simulink model "transystem2_testcase_5"  (R2019b)
settings: Solver=ode15s  StartTime=0.0  StopTime=1  RelTol=1e-3  AbsTol=1e-6
libraries: powerlib x48
settings Model: ExtModeTrigMode=oneshot  ExtModeArmWhenConnect=off  Creator=Dr. Lotfifard  LastModifiedBy=RAMYA
settings SolverCC: AutoScaleAbsTol=off
settings DataIOCC: SaveFormat=Array  SignalLoggingSaveFormat=ModelDataLogs  ReturnWorkspaceOutputs=off
settings OptimizationCC: BlockReduction=off  BooleanDataType=off  ExpressionDepthLimit=2147483647  LifeSpan=inf
settings DebuggingCC: SaveWithParameterizedLinksMsg=none  UnderspecifiedInitializationDetection=Classic  MergeDetectMultiDrivingBlocksExec=none  SignalResolutionControl=TryResolveAllWithWarning  MultiTaskDSMMsg=warning  MultiTaskCondExecSysMsg=none  FcnCallInpInsideContextMsg=warning  StateNameClashWarn=warning  SFUnexpectedBacktrackingDiag=warning  SFNoUnconditionalDefaultTransitionDiag=warning  SFExecutionAtInitializationDiag=none  ArithmeticOperatorsInVariantConditions=warning
settings HardwareCC: ProdBitPerPointer=32  ProdBitPerSizeT=32  ProdBitPerPtrDiffT=32  ProdLargestAtomicFloat=None  ProdIntDivRoundTo=Undefined  ProdEndianess=Unspecified  ProdWordSize=32  ProdHWDeviceType=32-bit Generic  TargetUnknown=on
settings ModelReferenceCC: PropagateSignalLabelsOutOfModel=off
settings SFSimCC: SimUseLocalCustomCode=off  CustomCodeUndefinedFunction=UseInterfaceOnly
settings RTWCC: RTWUseLocalCustomCode=off
settings CodeAppCC: StateflowObjectComments=on
settings GRTTargetCC: TargetLangStandard=C89/C90 (ANSI)  GeneratePreprocessorConditionals=Disable all  CombineOutputUpdateFcns=off  GRTInterface=on
settings ConfigComp: CovMetricSettings=dw  CovHtmlReporting=on  CovSaveCumulativeToWorkspaceVar=on  CovSaveSingleToWorkspaceVar=on  CovExternalEMLEnable=off
settings SimscapeCC: SimscapeNormalizeSystem=off

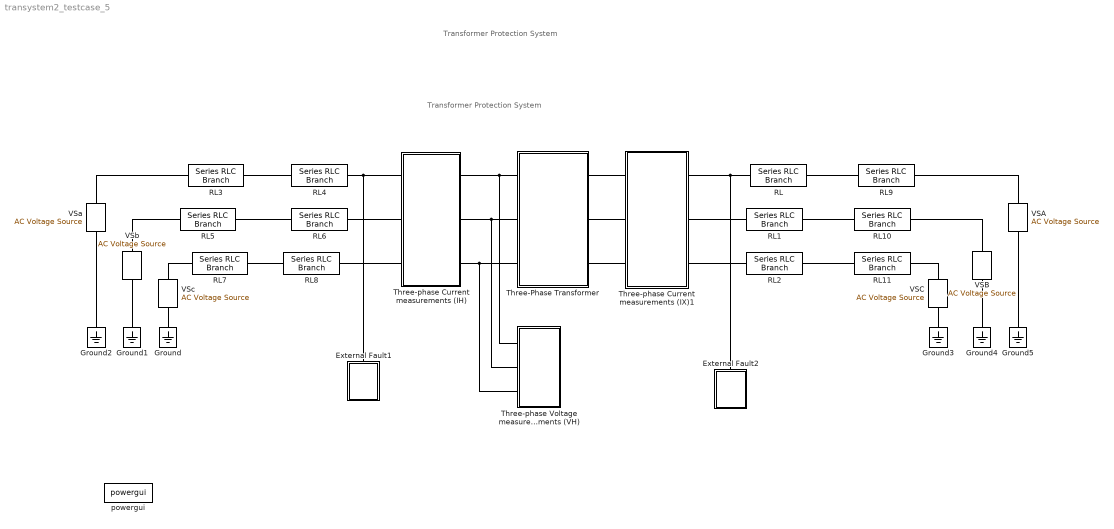
== system transystem2_testcase_5 ==
  note: Transformer Protection System
  note: Transformer Protection System
  External Fault1 : Subsystem  mask(Fault){RF=1, tf=1}
      mask prompts: RF "Resistance [ohm]"; tf "Time [sec]"
      mask Display: plot(0,0,100,100,[44,47,56,38,50],[23,8,64,44,97],[56,47],[25,8])
  External Fault2 : Subsystem  mask(Fault){RF=1, tf=1}
      mask prompts: RF "Resistance [ohm]"; tf "Time [sec]"
      mask Display: plot(0,0,100,100,[44,47,56,38,50],[23,8,64,44,97],[56,47],[25,8])
  Ground{,1..5} (6 alike) : powerlib/Elements/Ground  LConnTagsString=a
      settings: SourceProductName=Simscape Electrical
  RL{,1..11} (12 alike) : powerlib/Elements/Series RLC Branch  LConnTagsString=__new0  RConnTagsString=__new0  BranchType=RL  Resistance=50  Inductance=0.05  SetiL0=off  InitialCurrent=0  Capacitance=1e-6  Setx0=off  InitialVoltage=0  Measurements=None
      settings: SourceProductName=Simscape Electrical
  Three-Phase Transformer : Subsystem
  Three-phase Current measurements (IH) : Subsystem
  Three-phase Current measurements (IX)1 : Subsystem
  Three-phase Voltage measurements (VH) : Subsystem
  VSA : powerlib/Electrical Sources/AC Voltage Source  Amplitude=3.8e3/sqrt(3)*sqrt(2)  Phase=0  Frequency=60  SampleTime=0  Measurements=None  BusType=swing  Pref=10e3  Qref=0  Qmin=-inf  Qmax=+inf
      settings: SourceProductName=Simscape Electrical
  VSB : powerlib/Electrical Sources/AC Voltage Source  Amplitude=3.8e3/sqrt(3)*sqrt(2)  Phase=-120  Frequency=60  SampleTime=0  Measurements=None  BusType=swing  Pref=10e3  Qref=0  Qmin=-inf  Qmax=+inf
      settings: SourceProductName=Simscape Electrical
  VSC : powerlib/Electrical Sources/AC Voltage Source  Amplitude=3.8e3/sqrt(3)*sqrt(2)  Phase=120  Frequency=60  SampleTime=0  Measurements=None  BusType=swing  Pref=10e3  Qref=0  Qmin=-inf  Qmax=+inf
      settings: SourceProductName=Simscape Electrical
  VSa : powerlib/Electrical Sources/AC Voltage Source  Amplitude=315e3/sqrt(3)*sqrt(2)  Phase=0  Frequency=60  SampleTime=0  Measurements=None  BusType=swing  Pref=10e3  Qref=0  Qmin=-inf  Qmax=+inf
      settings: SourceProductName=Simscape Electrical
  VSb : powerlib/Electrical Sources/AC Voltage Source  Amplitude=315e3/sqrt(3)*sqrt(2)  Phase=-120  Frequency=60  SampleTime=0  Measurements=None  BusType=swing  Pref=10e3  Qref=0  Qmin=-inf  Qmax=+inf
      settings: SourceProductName=Simscape Electrical
  VSc : powerlib/Electrical Sources/AC Voltage Source  Amplitude=315e3/sqrt(3)*sqrt(2)  Phase=120  Frequency=60  SampleTime=0  Measurements=None  BusType=swing  Pref=10e3  Qref=0  Qmin=-inf  Qmax=+inf
      settings: SourceProductName=Simscape Electrical
  powergui : powerlib/powergui  SimulationMode=Continuous  SampleTime=0  frequency=60  Iterations=50  frequencyindice=60  Pbase=100e6  ErrMax=1e-4  UnitsV=kV  UnitsW=MW  buscounter=0  FunctionMessages=off  echomessages=off  EnableUseOfTLC=off  CurrentSourceSwitches=on  DisableSnubberDevices=off  DisableRonSwitches=off  DisableVfSwitches=off  DisplayEquations=off  AutomaticDiscreteSolvers=off  SolverType=Tustin/Backward Euler (TBE)  Interpol=off  ExternalGateDelay=off  methode=off  Ts=0  x0status=blocks  SPID=off  SwTol=0  HookPort=off  NonlinearTolerance=0  nMaxIteration=15  ContinueOnMaxIteration=off  RestoreLinks=warning  ResistiveCurrentMeasurement=off  Frange=[0:2:500]  Ylog=off  Xlog=on  ShowGrid=off  save=off  variable=ZData  structure=0  ZoomFFT=on  StartTime=0.0  cycles=1  DisplayStyle=1  fundamental=60  FreqAxis=off  MaxFrequency=1000  frequencyindicesteady=1  RmsSteady=1  display=off
      settings: SourceProductName=Simscape Electrical
  connections:
  Three-phase Current measurements (IH)/RConn2 -- Three-Phase Transformer/LConn2 -- Three-phase Voltage measurements (VH)/LConn2
  Three-Phase Transformer/LConn3 -- Three-phase Current measurements (IH)/RConn3 -- Three-phase Voltage measurements (VH)/LConn3
  RL/RConn1 -- RL9/LConn1
  RL3/RConn1 -- RL4/LConn1
  Three-phase Current measurements (IH)/RConn1 -- Three-Phase Transformer/LConn1 -- Three-phase Voltage measurements (VH)/LConn1
  Three-phase Current measurements (IH)/LConn1 -- External Fault1/LConn1 -- RL4/RConn1
  Ground/LConn1 -- VSc/LConn1
  RL10/RConn1 -- VSB/RConn1
  RL7/LConn1 -- VSc/RConn1
  RL9/RConn1 -- VSA/RConn1
  VSa/LConn1 -- Ground2/LConn1
  VSA/LConn1 -- Ground5/LConn1
  Three-phase Current measurements (IX)1/RConn3 -- RL2/LConn1
  RL6/LConn1 -- RL5/RConn1
  RL10/LConn1 -- RL1/RConn1
  Ground4/LConn1 -- VSB/LConn1
  Ground1/LConn1 -- VSb/LConn1
  Three-phase Current measurements (IX)1/RConn2 -- RL1/LConn1
  Three-Phase Transformer/RConn3 -- Three-phase Current measurements (IX)1/LConn3
  Three-Phase Transformer/RConn1 -- Three-phase Current measurements (IX)1/LConn1
  Three-phase Current measurements (IH)/LConn3 -- RL8/RConn1
  VSa/RConn1 -- RL3/LConn1
  Three-phase Current measurements (IH)/LConn2 -- RL6/RConn1
  RL5/LConn1 -- VSb/RConn1
  Three-phase Current measurements (IX)1/RConn1 -- External Fault2/LConn1 -- RL/LConn1
  RL11/RConn1 -- VSC/RConn1
  RL7/RConn1 -- RL8/LConn1
  Ground3/LConn1 -- VSC/LConn1
  RL2/RConn1 -- RL11/LConn1
  Three-Phase Transformer/RConn2 -- Three-phase Current measurements (IX)1/LConn2

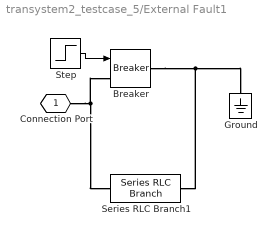
== system transystem2_testcase_5/External Fault1 ==
  Breaker : powerlib/Elements/Breaker  Tag=PoWeRsYsTeMbLoCk  InitialState=0  SwitchingTimes="[ 1/60  5/60 ]"  External=on  BreakerResistance=0.01  SnubberResistance=1e6  SnubberCapacitance=inf  Measurements=None  MoreParameters=off  NoBreakLoop=off
      settings: SourceProductName=Simscape Electrical
  Ground : powerlib/Elements/Ground  LConnTagsString=a
      settings: SourceProductName=Simscape Electrical
  Series RLC Branch1 : powerlib/Elements/Series RLC Branch  LConnTagsString=__new0  RConnTagsString=__new0  BranchType=RLC  Resistance=1  Inductance=1e-3  SetiL0=off  InitialCurrent=0  Capacitance=1e-6  Setx0=off  InitialVoltage=0  Measurements=None
      settings: SourceProductName=Simscape Electrical
  Step : Step  Time=tf
  Connection Port : PMIOPort  Tag=PMCPort  Side=Left
  wires:
  Step/1 -> Breaker/1
  connections:
  Breaker/RConn1 -- Ground/LConn1 -- Series RLC Branch1/RConn1
  Connection Port/RConn1 -- Breaker/LConn1 -- Series RLC Branch1/LConn1

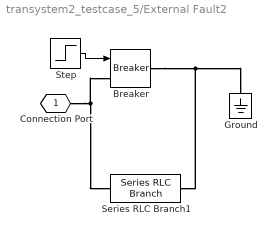
== system transystem2_testcase_5/External Fault2 ==
  Breaker : powerlib/Elements/Breaker  Tag=PoWeRsYsTeMbLoCk  InitialState=0  SwitchingTimes="[ 1/60  5/60 ]"  External=on  BreakerResistance=0.01  SnubberResistance=1e6  SnubberCapacitance=inf  Measurements=None  MoreParameters=off  NoBreakLoop=off
      settings: SourceProductName=Simscape Electrical
  Ground : powerlib/Elements/Ground  LConnTagsString=a
      settings: SourceProductName=Simscape Electrical
  Series RLC Branch1 : powerlib/Elements/Series RLC Branch  LConnTagsString=__new0  RConnTagsString=__new0  BranchType=RLC  Resistance=1  Inductance=1e-3  SetiL0=off  InitialCurrent=0  Capacitance=1e-6  Setx0=off  InitialVoltage=0  Measurements=None
      settings: SourceProductName=Simscape Electrical
  Step : Step  Time=tf
  Connection Port : PMIOPort  Tag=PMCPort  Side=Left
  wires:
  Step/1 -> Breaker/1
  connections:
  Breaker/RConn1 -- Ground/LConn1 -- Series RLC Branch1/RConn1
  Connection Port/RConn1 -- Breaker/LConn1 -- Series RLC Branch1/LConn1

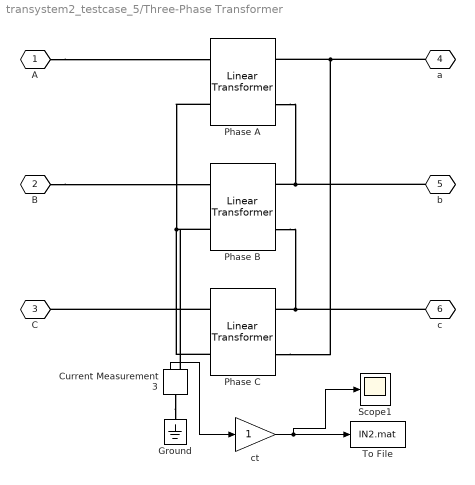
== system transystem2_testcase_5/Three-Phase Transformer ==
  Current Measurement3 : powerlib/Measurements/Current Measurement  PhasorSimulation=off  OutputType=Complex  PSBequivalent=0
      settings: SourceProductName=Simscape Electrical
  Ground : powerlib/Elements/Ground  LConnTagsString=a
      settings: SourceProductName=Simscape Electrical
  Phase A : powerlib/Elements/Linear Transformer  UNITS=pu  NominalPower=[ 300e6 60 ]  winding1="[ 315e3  0.0025  0.1 ]"  winding2="[ 13.8e3  0.0025  0.1 ]"  ThreeWindings=off  winding3=[ 315e3 0.002 0.08 ]  RmLm=[ 1e6 inf ]  Measurements=None  DataType=off
      settings: SourceProductName=Simscape Electrical
  Phase B : powerlib/Elements/Linear Transformer  UNITS=pu  NominalPower=[ 300e6 60 ]  winding1="[ 315e3  0.0025  0.1 ]"  winding2="[ 13.8e3  0.0025  0.1 ]"  ThreeWindings=off  winding3=[ 315e3 0.002 0.08 ]  RmLm=[ 1e6 inf ]  Measurements=None  DataType=off
      settings: SourceProductName=Simscape Electrical
  Phase C : powerlib/Elements/Linear Transformer  UNITS=pu  NominalPower=[ 300e6 60 ]  winding1="[ 315e3  0.0025  0.1 ]"  winding2="[ 13.8e3  0.0025  0.1 ]"  ThreeWindings=off  winding3=[ 315e3 0.002 0.08 ]  RmLm=[ 1e6 inf ]  Measurements=None  DataType=off
      settings: SourceProductName=Simscape Electrical
  Scope1 : Scope
  To File : ToFile  Filename=IN2.mat  MatrixName=iha
  ct : Gain  SaturateOnIntegerOverflow=on  OutDataTypeStr=Inherit: Same as input  ParamDataTypeStr=Inherit: Same as input
  A : PMIOPort  Tag=PMCPort  Side=Left
  B : PMIOPort  Tag=PMCPort  Port=2  Side=Left
  C : PMIOPort  Tag=PMCPort  Port=3  Side=Left
  a : PMIOPort  Tag=PMCPort  Port=4  Side=Right
  b : PMIOPort  Tag=PMCPort  Port=5  Side=Right
  c : PMIOPort  Tag=PMCPort  Port=6  Side=Right
  wires:
  ct/1 -> Scope1/1, To File/1
  Current Measurement3/1 -> ct/1
  connections:
  b/RConn1 -- Phase A/RConn2 -- Phase B/RConn1
  c/RConn1 -- Phase B/RConn2 -- Phase C/RConn1
  Phase B/LConn2 -- Current Measurement3/RConn1 -- Phase C/LConn2 -- Phase A/LConn2
  a/RConn1 -- Phase C/RConn2 -- Phase A/RConn1
  A/RConn1 -- Phase A/LConn1
  Current Measurement3/LConn1 -- Ground/LConn1
  Phase C/LConn1 -- C/RConn1
  B/RConn1 -- Phase B/LConn1

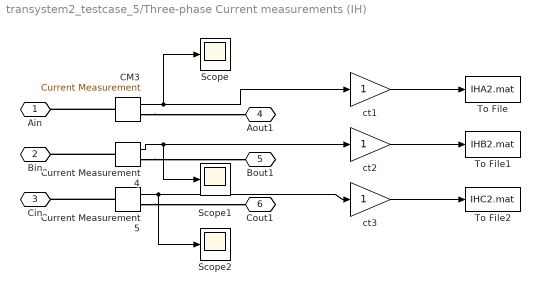
== system transystem2_testcase_5/Three-phase Current measurements (IH) ==
  CM3 : powerlib/Measurements/Current Measurement  PhasorSimulation=off  OutputType=Complex  PSBequivalent=0
      settings: SourceProductName=Simscape Electrical
  Current Measurement4 : powerlib/Measurements/Current Measurement  PhasorSimulation=off  OutputType=Complex  PSBequivalent=0
      settings: SourceProductName=Simscape Electrical
  Current Measurement5 : powerlib/Measurements/Current Measurement  PhasorSimulation=off  OutputType=Complex  PSBequivalent=0
      settings: SourceProductName=Simscape Electrical
  Scope : Scope
  Scope1 : Scope
  Scope2 : Scope
  To File : ToFile  Filename=IHA2.mat  MatrixName=iha
  To File1 : ToFile  Filename=IHB2.mat  MatrixName=ihb
  To File2 : ToFile  Filename=IHC2.mat  MatrixName=ihc
  ct1 : Gain  SaturateOnIntegerOverflow=on  OutDataTypeStr=Inherit: Same as input  ParamDataTypeStr=Inherit: Same as input
  ct2 : Gain  SaturateOnIntegerOverflow=on  OutDataTypeStr=Inherit: Same as input  ParamDataTypeStr=Inherit: Same as input
  ct3 : Gain  SaturateOnIntegerOverflow=on  OutDataTypeStr=Inherit: Same as input  ParamDataTypeStr=Inherit: Same as input
  Ain : PMIOPort  Side=Left
  Bin : PMIOPort  Port=2  Side=Left
  Cin : PMIOPort  Port=3  Side=Left
  Aout1 : PMIOPort  Port=4  Side=Right
  Bout1 : PMIOPort  Port=5  Side=Right
  Cout1 : PMIOPort  Port=6  Side=Right
  wires:
  ct2/1 -> To File1/1
  ct3/1 -> To File2/1
  Current Measurement4/1 -> Scope1/1, ct2/1
  CM3/1 -> Scope/1, ct1/1
  Current Measurement5/1 -> Scope2/1, ct3/1
  ct1/1 -> To File/1
  connections:
  Current Measurement4/RConn1 -- Bout1/RConn1
  CM3/LConn1 -- Ain/RConn1
  Current Measurement5/LConn1 -- Cin/RConn1
  CM3/RConn1 -- Aout1/RConn1
  Current Measurement4/LConn1 -- Bin/RConn1
  Current Measurement5/RConn1 -- Cout1/RConn1

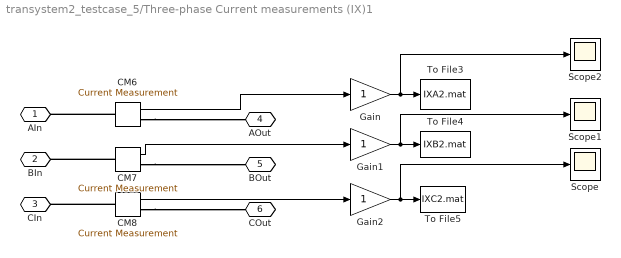
== system transystem2_testcase_5/Three-phase Current measurements (IX)1 ==
  CM6 : powerlib/Measurements/Current Measurement  PhasorSimulation=off  OutputType=Complex  PSBequivalent=0
      settings: SourceProductName=Simscape Electrical
  CM7 : powerlib/Measurements/Current Measurement  PhasorSimulation=off  OutputType=Complex  PSBequivalent=0
      settings: SourceProductName=Simscape Electrical
  CM8 : powerlib/Measurements/Current Measurement  PhasorSimulation=off  OutputType=Complex  PSBequivalent=0
      settings: SourceProductName=Simscape Electrical
  Gain : Gain  SaturateOnIntegerOverflow=on  OutDataTypeStr=Inherit: Same as input  ParamDataTypeStr=Inherit: Same as input
  Gain1 : Gain  SaturateOnIntegerOverflow=on  OutDataTypeStr=Inherit: Same as input  ParamDataTypeStr=Inherit: Same as input
  Gain2 : Gain  SaturateOnIntegerOverflow=on  OutDataTypeStr=Inherit: Same as input  ParamDataTypeStr=Inherit: Same as input
  Scope : Scope
  Scope1 : Scope
  Scope2 : Scope
  To File3 : ToFile  Filename=IXA2.mat  MatrixName=ixa
  To File4 : ToFile  Filename=IXB2.mat  MatrixName=ixb
  To File5 : ToFile  Filename=IXC2.mat  MatrixName=ixc
  AIn : PMIOPort  Side=Left
  BIn : PMIOPort  Port=2  Side=Left
  CIn : PMIOPort  Port=3  Side=Left
  AOut : PMIOPort  Port=4  Side=Right
  BOut : PMIOPort  Port=5  Side=Right
  COut : PMIOPort  Port=6  Side=Right
  wires:
  Gain2/1 -> To File5/1, Scope/1
  Gain1/1 -> To File4/1, Scope1/1
  Gain/1 -> To File3/1, Scope2/1
  CM7/1 -> Gain1/1
  CM6/1 -> Gain/1
  CM8/1 -> Gain2/1
  connections:
  CM7/RConn1 -- BOut/RConn1
  CM6/LConn1 -- AIn/RConn1
  CM6/RConn1 -- AOut/RConn1
  CM8/RConn1 -- COut/RConn1
  CM7/LConn1 -- BIn/RConn1
  CM8/LConn1 -- CIn/RConn1

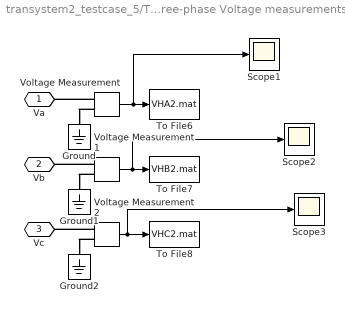
== system transystem2_testcase_5/Three-phase Voltage measurements (VH) ==
  Ground : powerlib/Elements/Ground  LConnTagsString=a
      settings: SourceProductName=Simscape Electrical
  Ground1 : powerlib/Elements/Ground  LConnTagsString=a
      settings: SourceProductName=Simscape Electrical
  Ground2 : powerlib/Elements/Ground  LConnTagsString=a
      settings: SourceProductName=Simscape Electrical
  Scope1 : Scope
  Scope2 : Scope
  Scope3 : Scope
  To File6 : ToFile  Filename=VHA2.mat  MatrixName=vha
  To File7 : ToFile  Filename=VHB2.mat  MatrixName=vhb
  To File8 : ToFile  Filename=VHC2.mat  MatrixName=vhc
  Voltage Measurement : powerlib/Measurements/Voltage Measurement  PhasorSimulation=off  OutputType=Complex  PSBequivalent=0
      settings: SourceProductName=Simscape Electrical
  Voltage Measurement1 : powerlib/Measurements/Voltage Measurement  PhasorSimulation=off  OutputType=Complex  PSBequivalent=0
      settings: SourceProductName=Simscape Electrical
  Voltage Measurement2 : powerlib/Measurements/Voltage Measurement  PhasorSimulation=off  OutputType=Complex  PSBequivalent=0
      settings: SourceProductName=Simscape Electrical
  Va : PMIOPort  Side=Left
  Vb : PMIOPort  Port=2  Side=Left
  Vc : PMIOPort  Port=3  Side=Left
  wires:
  Voltage Measurement/1 -> Scope1/1, To File6/1
  Voltage Measurement1/1 -> Scope2/1, To File7/1
  Voltage Measurement2/1 -> Scope3/1, To File8/1
  connections:
  Voltage Measurement/LConn2 -- Ground/LConn1
  Voltage Measurement1/LConn2 -- Ground1/LConn1
  Voltage Measurement2/LConn2 -- Ground2/LConn1
  Voltage Measurement2/LConn1 -- Vc/RConn1
  Voltage Measurement1/LConn1 -- Vb/RConn1
  Voltage Measurement/LConn1 -- Va/RConn1
